simulink model "Transitions2_2018a"  (R2018a)
settings: Solver=VariableStepAuto  StartTime=0.0  StopTime=0.2  RelTol=1e-3
settings Model: Creator=BEAR  LastModifiedBy=bzhan

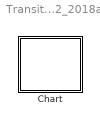
== system Transitions2_2018a ==
  Chart : Stateflow chart  TreatAsAtomicUnit=on

== stateflow chart Transitions2_2018a/Chart ==
  settings: updateMethod=DISCRETE  sampleTime=0.1
  state S
    en: f("enS")
    ex: f("exS")
    state A
      en: f("enA")
      ex: f("exA")
    state B
      en: f("enB")
      ex: f("exB")
    (default) -> A
    A -> B
  state T
    en: f("enT")
    ex: f("exT")
    state C
      en: f("enB")
      ex: f("exB")
    (default) -> C
  (default) -> S
  B -> T : {f("ca")}/{f("ta")}
  data: s function_input
  function f(s):
    | function f(s)
    |   fprintf(s+"\n");
